simulink model "ProjectSimControl"  (R2022b)
settings: Solver=FixedStepAuto  StartTime=0.0  StopTime=tspan  FixedStep=10  RelTol=1e-3
values from neighbouring files (symbols this model uses):
  E_b_ECI_0 = C2EulerAngles(C_b_ECI_0)    [A421_FinalProject_Pt5.m]    (also in A421_FinalProject_Pt6.m; Final_Project_Part_3_disturbances.m; Final_Project_Part_3_disturbances_init_Template-1.m; Final_Project_Part_3_disturbances_init_Template.m)
  J = [812.04 0 0; 0 545.37 0; 0 0 627.71]    [A421_FinalProject_Pt5.m]    (also in A421_FinalProject_Pt6.m; Final_Project_Part_3_disturbances_torques.m; Final_Project_Pt4.m; hw5.m = diag([1200, 2000, 2800]))
  q_b_ECI_0 = C2quat(C_b_ECI_0)    [A421_FinalProject_Pt5.m]    (also in A421_FinalProject_Pt6.m = [epsilon_b_ECI_0; sqrt(1-norm(epsilon_b_ECI_0)^2)]; Final_Project_Part_3_disturbances.m; Final_Project_Part_3_disturbances_init_Template-1.m; Final_Project_Part_3_disturbances_init_Template.m)
  T = [0;0;0]    [A421_FinalProject_Pt6.m]    (also in hw5.m; main.m)
  w_b_ECI_0 = [0.001; -0.001; 0.002]    [A421_FinalProject_Pt5.m]    (also in A421_FinalProject_Pt6.m; Final_Project_Part_3_disturbances.m; Final_Project_Part_3_disturbances_init_Template-1.m; Final_Project_Part_3_disturbances_init_Template.m)
settings Model: Creator=emehiel  LastModifiedBy=ryanp
settings SolverCC: AlgebraicLoopSolver=TrustRegion
settings DebuggingCC: UnconnectedInputMsg=warning  UnconnectedOutputMsg=warning  UnconnectedLineMsg=warning  SFMachineParentedDataDiag=warning
settings ModelReferenceCC: EnableRefExpFcnMdlSchedulingChecks=on

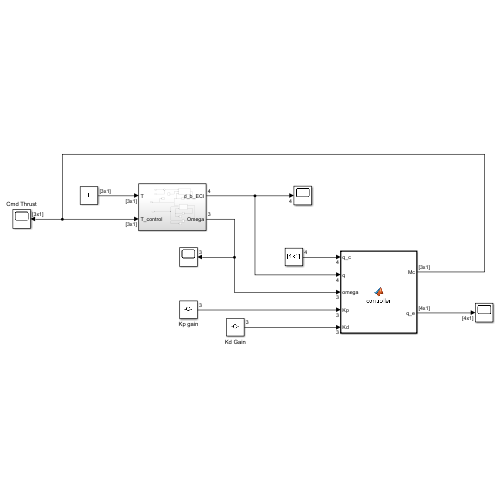
[thumbnail: Simulink's stored preview of the top-level diagram]
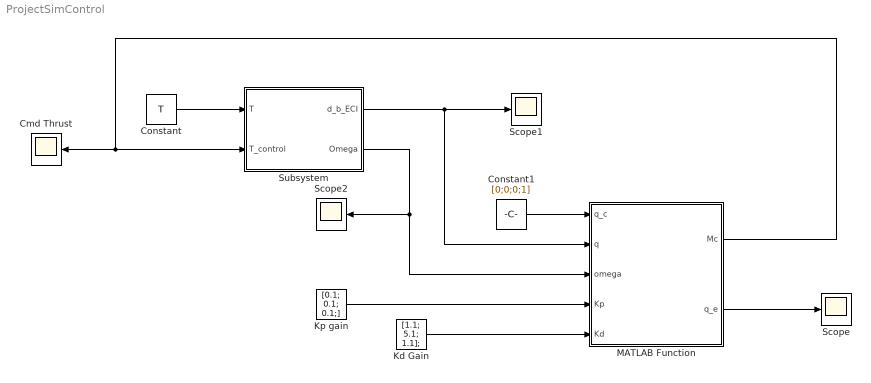
== system ProjectSimControl ==
  Cmd Thrust : Scope
  Constant : Constant  Value=T  VectorParams1D=off
  Constant1 : Constant  Value=[0;0;0;1]
  Kd Gain : Constant  Value=[1.1; 5.1; 1.1];
  Kp gain : Constant  Value=[0.1; 0.1; 0.1;]
  MATLAB Function : MATLAB Function  TreatAsAtomicUnit=on
  Scope : Scope
  Scope1 : Scope
  Scope2 : Scope
  Subsystem : Subsystem
  wires:
  Kd Gain/1 -> MATLAB Function/5(Kd)
  Kp gain/1 -> MATLAB Function/4(Kp)
  Subsystem/1(d_b_ECI) -> Scope1/1, MATLAB Function/2(q)
  Subsystem/2(Omega) -> Scope2/1, MATLAB Function/3(omega)
  Constant/1 -> Subsystem/1(T)
  MATLAB Function/2(q_e) -> Scope/1
  Constant1/1 -> MATLAB Function/1(q_c)
  MATLAB Function/1(Mc) -> Subsystem/2(T_control), Cmd Thrust/1

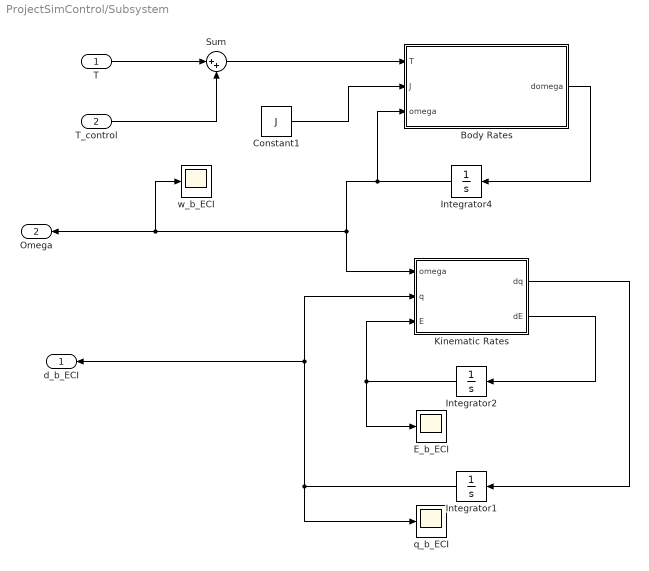
== system ProjectSimControl/Subsystem ==
  T : Inport
  T_control : Inport  Port=2
  Body Rates : MATLAB Function  TreatAsAtomicUnit=on
  Constant1 : Constant  Value=J
  E_b_ECI : Scope
  Integrator1 : Integrator  InitialCondition=q_b_ECI_0
  Integrator2 : Integrator  InitialCondition=E_b_ECI_0
  Integrator4 : Integrator  InitialCondition=w_b_ECI_0
  Kinematic Rates : MATLAB Function  TreatAsAtomicUnit=on
  Sum : Sum  Inputs=|++
  q_b_ECI : Scope
  w_b_ECI : Scope
  d_b_ECI : Outport
  Omega : Outport  Port=2
  wires:
  Kinematic Rates/2(dE) -> Integrator2/1
  Integrator2/1 -> Kinematic Rates/3(E), E_b_ECI/1
  Kinematic Rates/1(dq) -> Integrator1/1
  Integrator1/1 -> Kinematic Rates/2(q), d_b_ECI/1, q_b_ECI/1
  Body Rates/1(domega) -> Integrator4/1
  Integrator4/1 -> Omega/1, w_b_ECI/1, Kinematic Rates/1(omega), Body Rates/3(omega)
  Constant1/1 -> Body Rates/2(J)
  T/1 -> Sum/1
  Sum/1 -> Body Rates/1(T)
  T_control/1 -> Sum/2

== matlab function ProjectSimControl/MATLAB Function ==
  data: q_c input; Mc output; q input; omega input; Kp input; Kd input; q_e output
function [Mc, q_e] = controller(q_c, q, omega, Kp, Kd)
% q_e = quatMult(q, quatConjugate(q_c));
% Compute the conjugate of q_c
q_c_conj = [q_c(1), -q_c(2), -q_c(3), -q_c(4)];

% Compute the quaternion multiplication q * q_c_conj
q0 = q(1); q1 = q(2); q2 = q(3); q3 = q(4);
p0 = q_c_conj(1); p1 = q_c_conj(2); p2 = q_c_conj(3); p3 = q_c_conj(4);
q1 = q0 * p0 - q1 * p1 - q2 * p2 - q3 * p3;
q2 = q0 * p1 + q1 * p0 + q2 * p3 - q3 * p2;
q3 = q0 * p2 - q1 * p3 + q2 * p0 + q3 * p1;
q4 = q0 * p3 + q1 * p2 - q2 * p1 + q3 * p0;

q_e = [q1; q2; q3; q4];


Mc = -Kp.*q_e(2:4) - Kd.*omega;

== matlab function ProjectSimControl/Subsystem/Kinematic Rates ==
  data: omega input; q input; dq output; E input; dE output
function [dq,dE] = kinematics(omega, q, E)
%#codegen

I = eye(3); %Identity

% unpack quaternion
eps1 = q(1);
eps2 = q(2);
eps3 = q(3);
eps = [eps1; eps2; eps3];

eda = q(4);

% compute the derivative of the quaternion components here
             
%Quaternion rates Eq.1.56
eps_cross = [0,  -eps3, eps2;
             eps3,  0, -eps1;
             -eps2, eps1, 0];

deps = 0.5*(eda*I + eps_cross)*omega;
deda = -0.5*eps'*omega;

dq = [deps; deda];

% compute the derivative of the Euler Angle components here
            
%Euler rates
phi = E(1);
theta = E(2);
R = [1 sin(phi)*tan(theta) cos(phi)*tan(theta);
     0     cos(phi)           -sin(phi);
     0 sin(phi)*sec(theta) cos(phi)*sec(theta)];
    
dE = R*omega;


end

== matlab function ProjectSimControl/Subsystem/Body Rates ==
  data: T input; J input; omega input; domega output
function domega = dynamics(T, J, omega)
%#codegen


% Compute the derivative of the angular velocity $\omega$ here

domega = J \ (T - cross(-omega, J*omega));

% phi = omega(1);
% theta = omega(2);
% psi = omega(3);
% 
% %From body to euler rates
% matrix = [1 sin(phi)*tan(theta) cos(phi)*tan(theta);
%           0    cos(phi)            -sin(phi);
%           0 sin(phi)*sec(theta) cos(phi)*sec(theta)];
% 
% domega = matrix * omega;

end
